simulink model "untitled"  (R2024b)
settings: Solver=VariableStepAuto  StartTime=0.0  StopTime=100  RelTol=1e-3
settings Model: Creator=robin  LastModifiedBy=robin

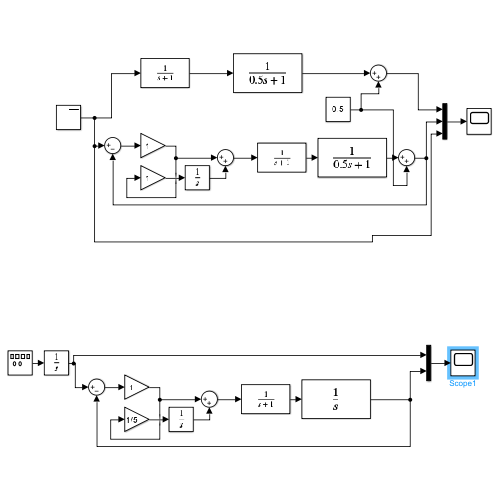
[thumbnail: Simulink's stored preview of the top-level diagram]
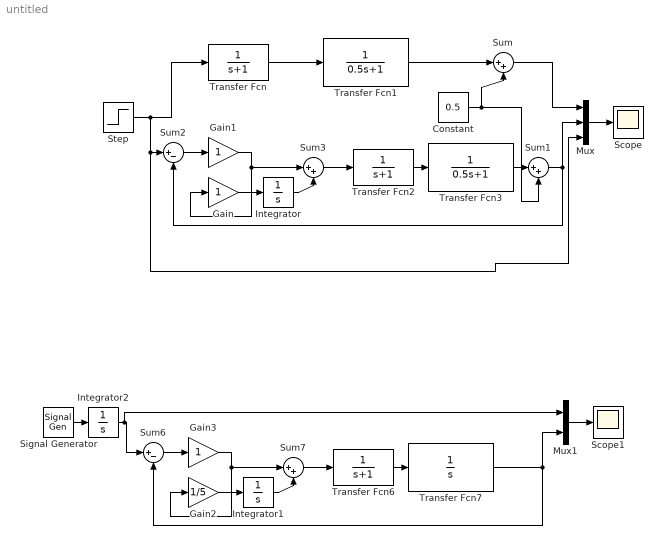
== system untitled ==
  Constant : Constant  Value=0.5
  Gain : Gain
  Gain1 : Gain
  Gain2 : Gain  Gain=1/5
  Gain3 : Gain
  Integrator : Integrator
  Integrator1 : Integrator
  Integrator2 : Integrator
  Mux : Mux  Inputs=3
  Mux1 : Mux  Inputs=2
  Scope : Scope
  Scope1 : Scope
  Signal Generator : SignalGenerator  WaveForm=square  Amplitude=0.2  Frequency=0.2  Units=rad/sec
  Step : Step  Time=5  SampleTime=0
  Sum{,1,3,7} (4 alike) : Sum  Inputs=|++
  Sum2 : Sum  Inputs=|+-
  Sum6 : Sum  Inputs=|+-
  Transfer Fcn : TransferFcn  Denominator=[1 1]
  Transfer Fcn1 : TransferFcn  Denominator=[0.5 1]
  Transfer Fcn2 : TransferFcn  Denominator=[1 1]
  Transfer Fcn3 : TransferFcn  Denominator=[0.5 1]
  Transfer Fcn6 : TransferFcn  Denominator=[1 1]
  Transfer Fcn7 : TransferFcn  Denominator=[1 0]
  wires:
  Step/1 -> Sum2/1, Mux/3, Transfer Fcn/1
  Transfer Fcn/1 -> Transfer Fcn1/1
  Transfer Fcn1/1 -> Sum/1
  Constant/1 -> Sum1/2, Sum/2
  Transfer Fcn2/1 -> Transfer Fcn3/1
  Transfer Fcn3/1 -> Sum1/1
  Sum/1 -> Mux/1
  Sum1/1 -> Sum2/2, Mux/2
  Sum3/1 -> Transfer Fcn2/1
  Integrator/1 -> Sum3/2
  Gain/1 -> Integrator/1
  Sum2/1 -> Gain1/1
  Gain1/1 -> Sum3/1, Gain/1
  Mux/1 -> Scope/1
  Mux1/1 -> Scope1/1
  Gain3/1 -> Sum7/1, Gain2/1
  Integrator1/1 -> Sum7/2
  Gain2/1 -> Integrator1/1
  Sum6/1 -> Gain3/1
  Sum7/1 -> Transfer Fcn6/1
  Transfer Fcn6/1 -> Transfer Fcn7/1
  Transfer Fcn7/1 -> Sum6/2, Mux1/2
  Signal Generator/1 -> Integrator2/1
  Integrator2/1 -> Mux1/1, Sum6/1
